simulink model "WLTP"  (R2020b)
settings: Solver=FixedStepAuto  StartTime=0.0  StopTime=1800  FixedStep=1  RelTol=1e-3
values from neighbouring files (symbols this model uses):
  A = 2.4    [Ansteuerung_WLTP.m]
  cw = 0.28    [Ansteuerung_WLTP.m]
  eta = VKM.eta    [Ansteuerung_WLTP.m]
  eta_diff = 0.99    [Ansteuerung_WLTP.m]
  eta_getr = 0.96    [Ansteuerung_WLTP.m]
  Fr = 40    [Ansteuerung_WLTP.m]
  fr = 1e-3    (= 0.001)    [Ansteuerung_WLTP.m]
  g = 9.81    [Ansteuerung_WLTP.m]
  i = [4.776 3.360 2.311 1.553 1.020 0.655]    [Ansteuerung_WLTP.m]
  i_AG = 3.825    [Ansteuerung_WLTP.m]
  lambda = 1.25    [Ansteuerung_WLTP.m]
  M_1 = eta_diff*eta_getr*VKM.full_load_M*i(1)*i_AG    [Ansteuerung_WLTP.m]
  M_2 = eta_diff*eta_getr*VKM.full_load_M*i(2)*i_AG    [Ansteuerung_WLTP.m]
  M_3 = eta_diff*eta_getr*VKM.full_load_M*i(3)*i_AG    [Ansteuerung_WLTP.m]
  M_4 = eta_diff*eta_getr*VKM.full_load_M*i(4)*i_AG    [Ansteuerung_WLTP.m]
  M_5 = eta_diff*eta_getr*VKM.full_load_M*i(5)*i_AG    [Ansteuerung_WLTP.m]
  M_6 = eta_diff*eta_getr*VKM.full_load_M*i(6)*i_AG    [Ansteuerung_WLTP.m]
  mfzg = 1500    [Ansteuerung_WLTP.m]
  mzul = 475    [Ansteuerung_WLTP.m]
  n_u = 900    [Ansteuerung_WLTP.m]
  rdyn = 0.35    [Ansteuerung_WLTP.m]
  rho = 1.2    [Ansteuerung_WLTP.m]
  v1_1 = (pi*VKM.full_load_n*rdyn)*3.6/(30*i_AG*i(1))    [Ansteuerung_WLTP.m]
  v1_2 = (pi*VKM.full_load_n*rdyn)*3.6/(30*i_AG*i(2))    [Ansteuerung_WLTP.m]
  v1_3 = (pi*VKM.full_load_n*rdyn)*3.6/(30*i_AG*i(3))    [Ansteuerung_WLTP.m]
  v1_4 = (pi*VKM.full_load_n*rdyn)*3.6/(30*i_AG*i(4))    [Ansteuerung_WLTP.m]
  v1_5 = (pi*VKM.full_load_n*rdyn)*3.6/(30*i_AG*i(5))    [Ansteuerung_WLTP.m]
  v1_6 = (pi*VKM.full_load_n*rdyn)*3.6/(30*i_AG*i(6))    [Ansteuerung_WLTP.m]
  VKM =     [VKM.mat]
  WLTP_t = [0:1800].'    [Ansteuerung_WLTP.m]
  WLTP_v = [0;0;0;0;0;0;0;0;0;0;0;0;0.200000000000000;1.70000000000000;5.40000000000000;9.90000000000000;13.1000000000000;16.9000000000000;21.7000000000000;26;27.5000000000000;28.1000000000000;28.3000000000000;28.8000000000000;29.1000000000000;30.8000000000000;31.9000000000000;34.1000000000000;36.6000000000000;39.1000000000000;41.3000000000000;42.5000000000000;43.3000000000000;43.9000000000000;44.40000000000 ...(+23900 chars)    [Ansteuerung_WLTP.m]
settings Model: Creator=ohms  LastModifiedBy=kusno

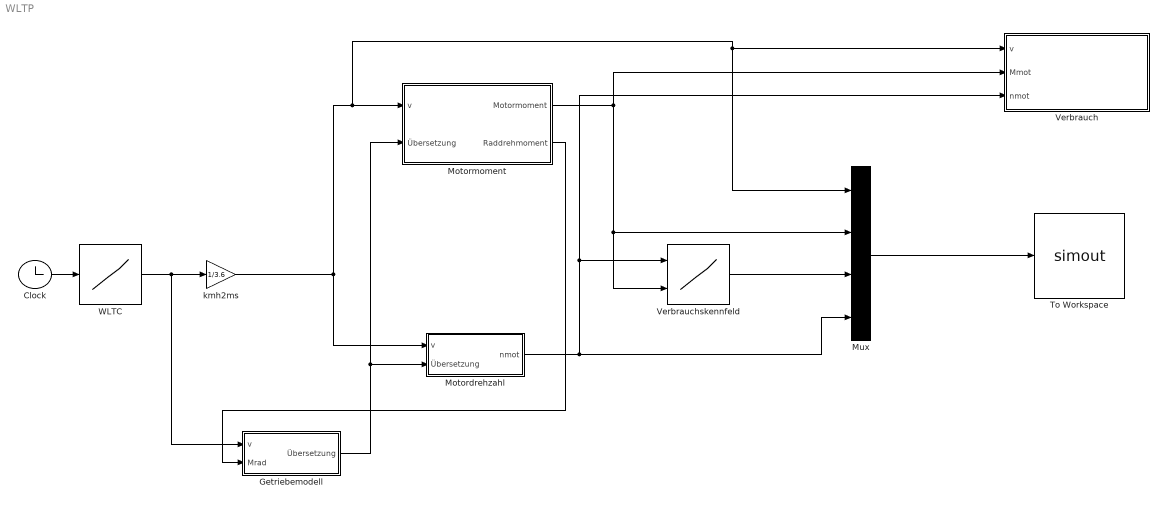
== system WLTP ==
  Clock : Clock
  Getriebemodell : Subsystem
  Motordrehzahl : Subsystem
  Motormoment : Subsystem
  Mux : Mux
  To Workspace : ToWorkspace  VariableName=simout  SaveFormat=Timeseries  SampleTime=-1
  Verbrauch : Subsystem
  Verbrauchskennfeld : Lookup_n-D  BreakpointsForDimension1=VKM.n_axis(:,1)  BreakpointsForDimension2=VKM.M_axis(1,:)  Table=eta  ExtrapMethod=Clip  InternalRulePriority=Speed  RndMeth=Simplest  InputSameDT=on
      settings: InputPortMap=u0,u1
  WLTC : Lookup_n-D  NumberOfTableDimensions=1  BreakpointsForDimension1=WLTP_t  Table=WLTP_v  InternalRulePriority=Speed  RndMeth=Simplest  InputSameDT=on
  kmh2ms : Gain  Gain=1/3.6
  wires:
  Clock/1 -> WLTC/1
  Getriebemodell/1(Übersetzung) -> Motormoment/2(Übersetzung), Motordrehzahl/2(Übersetzung)
  kmh2ms/1 -> Motormoment/1(v), Mux/1, Verbrauch/1(v), Motordrehzahl/1(v)
  Motordrehzahl/1(nmot) -> Verbrauch/3(nmot), Verbrauchskennfeld/1, Mux/4
  Mux/1 -> To Workspace/1
  Motormoment/1(Motormoment) -> Mux/2, Verbrauchskennfeld/2, Verbrauch/2(Mmot)
  Verbrauchskennfeld/1 -> Mux/3
  Motormoment/2(Raddrehmoment) -> Getriebemodell/2(Mrad)
  WLTC/1 -> Getriebemodell/1(v), kmh2ms/1

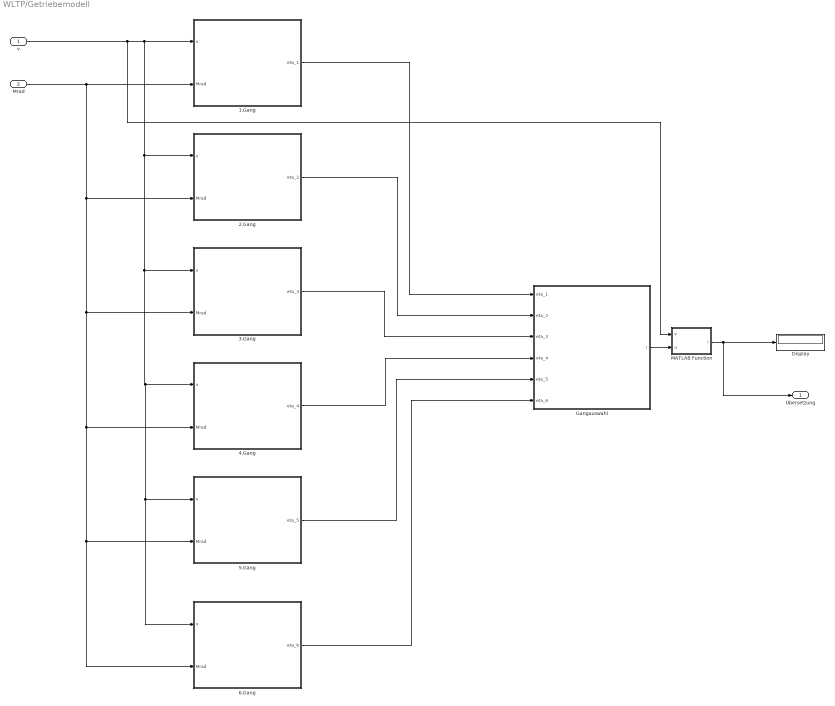
== system WLTP/Getriebemodell ==
  v : Inport
  Mrad : Inport  Port=2
  1.Gang : Subsystem
  2.Gang : Subsystem
  3.Gang : Subsystem
  4.Gang : Subsystem
  5.Gang : Subsystem
  6.Gang : Subsystem
  Display : Display
  Gangauswahl : MATLAB Function  TreatAsAtomicUnit=on
  MATLAB Function : MATLAB Function  TreatAsAtomicUnit=on
  Übersetzung : Outport
  wires:
  Mrad/1 -> 6.Gang/2(Mrad), 5.Gang/2(Mrad), 4.Gang/2(Mrad), 3.Gang/2(Mrad), 2.Gang/2(Mrad), 1.Gang/2(Mrad)
  1.Gang/1(eta_1) -> Gangauswahl/1(eta_1)
  2.Gang/1(eta_2) -> Gangauswahl/2(eta_2)
  3.Gang/1(eta_3) -> Gangauswahl/3(eta_3)
  4.Gang/1(eta_4) -> Gangauswahl/4(eta_4)
  5.Gang/1(eta_5) -> Gangauswahl/5(eta_5)
  6.Gang/1(eta_6) -> Gangauswahl/6(eta_6)
  Gangauswahl/1(i) -> MATLAB Function/2(u)
  MATLAB Function/1(i) -> Display/1, Übersetzung/1
  v/1 -> MATLAB Function/1(v), 6.Gang/1(v), 5.Gang/1(v), 4.Gang/1(v), 3.Gang/1(v), 2.Gang/1(v), 1.Gang/1(v)

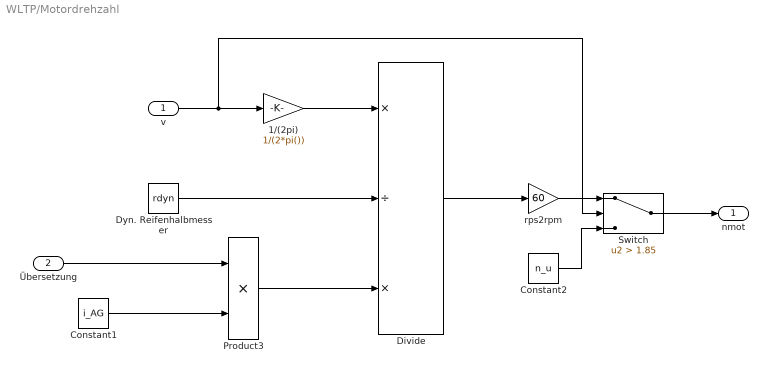
== system WLTP/Motordrehzahl ==
  v : Inport
  Übersetzung : Inport  Port=2
  1/(2pi) : Gain  Gain=1/(2*pi())
  Constant1 : Constant  Value=i_AG
  Constant2 : Constant  Value=n_u
  Divide : Product  Inputs=*/*
  Dyn. Reifenhalbmesser : Constant  Value=rdyn
  Product3 : Product
  Switch : Switch  Criteria=u2 > Threshold  Threshold=1.85
  rps2rpm : Gain  Gain=60
  nmot : Outport
  wires:
  v/1 -> Switch/2, 1/(2pi)/1
  1/(2pi)/1 -> Divide/1
  Dyn. Reifenhalbmesser/1 -> Divide/2
  Divide/1 -> rps2rpm/1
  Übersetzung/1 -> Product3/1
  Constant1/1 -> Product3/2
  Product3/1 -> Divide/3
  Switch/1 -> nmot/1
  rps2rpm/1 -> Switch/1
  Constant2/1 -> Switch/3

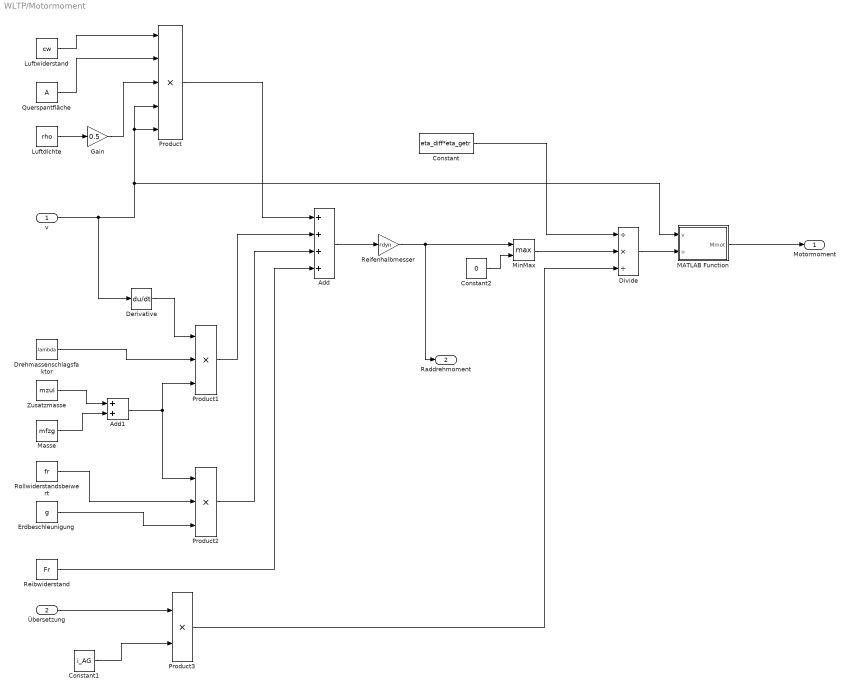
== system WLTP/Motormoment ==
  v : Inport
  Übersetzung : Inport  Port=2
  Add : Sum  Inputs=++++
  Add1 : Sum
  Constant : Constant  Value=eta_diff*eta_getr
  Constant1 : Constant  Value=i_AG
  Constant2 : Constant  Value=0
  Derivative : Derivative
  Divide : Product  Inputs=/*/
  Drehmassenschlagsfaktor : Constant  Value=lambda
  Erdbeschleunigung : Constant  Value=g
  Gain : Gain  Gain=0.5
  Luftdichte : Constant  Value=rho
  Luftwiderstand : Constant  Value=cw
  MATLAB Function : MATLAB Function  TreatAsAtomicUnit=on
  Masse : Constant  Value=mfzg
  MinMax : MinMax  Function=max  Inputs=2
  Product : Product  Inputs=5
  Product1 : Product  Inputs=3
  Product2 : Product  Inputs=3
  Product3 : Product
  Querspantfläche : Constant  Value=A
  Reibwiderstand : Constant  Value=Fr
  Reifenhalbmesser : Gain  Gain=rdyn
  Rollwiderstandsbeiwert : Constant  Value=fr
  Zusatzmasse : Constant  Value=mzul
  Motormoment : Outport
  Raddrehmoment : Outport  Port=2
  wires:
  Luftwiderstand/1 -> Product/1
  Querspantfläche/1 -> Product/2
  Luftdichte/1 -> Gain/1
  Gain/1 -> Product/3
  Derivative/1 -> Product1/1
  Drehmassenschlagsfaktor/1 -> Product1/2
  Rollwiderstandsbeiwert/1 -> Product2/2
  Erdbeschleunigung/1 -> Product2/3
  v/1 -> Derivative/1, MATLAB Function/1(v), Product/5, Product/4
  Product/1 -> Add/1
  Product1/1 -> Add/2
  Product2/1 -> Add/3
  Reifenhalbmesser/1 -> MinMax/1, Raddrehmoment/1
  Reibwiderstand/1 -> Add/4
  Constant/1 -> Divide/1
  Übersetzung/1 -> Product3/1
  Constant1/1 -> Product3/2
  Product3/1 -> Divide/3
  Add/1 -> Reifenhalbmesser/1
  Divide/1 -> MATLAB Function/2(u)
  MATLAB Function/1(Mmot) -> Motormoment/1
  Zusatzmasse/1 -> Add1/1
  Masse/1 -> Add1/2
  Add1/1 -> Product1/3, Product2/1
  MinMax/1 -> Divide/2
  Constant2/1 -> MinMax/2

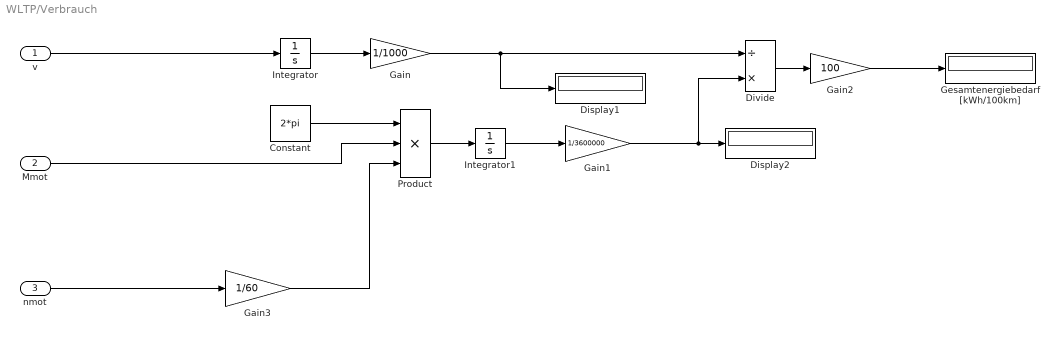
== system WLTP/Verbrauch ==
  v : Inport
  Mmot : Inport  Port=2
  nmot : Inport  Port=3
  Constant : Constant  Value=2*pi
  Display1 : Display
  Display2 : Display
  Divide : Product  Inputs=/*
  Gain : Gain  Gain=1/1000
  Gain1 : Gain  Gain=1/3600000
  Gain2 : Gain  Gain=100
  Gain3 : Gain  Gain=1/60
  Gesamtenergiebedarf [kWh/100km] : Display
  Integrator : Integrator
  Integrator1 : Integrator
  Product : Product  Inputs=3
  wires:
  Gain1/1 -> Display2/1, Divide/2
  Mmot/1 -> Product/2
  Integrator/1 -> Gain/1
  Divide/1 -> Gain2/1
  v/1 -> Integrator/1
  Gain/1 -> Display1/1, Divide/1
  Product/1 -> Integrator1/1
  Constant/1 -> Product/1
  nmot/1 -> Gain3/1
  Gain2/1 -> Gesamtenergiebedarf [kWh/100km]/1
  Integrator1/1 -> Gain1/1
  Gain3/1 -> Product/3

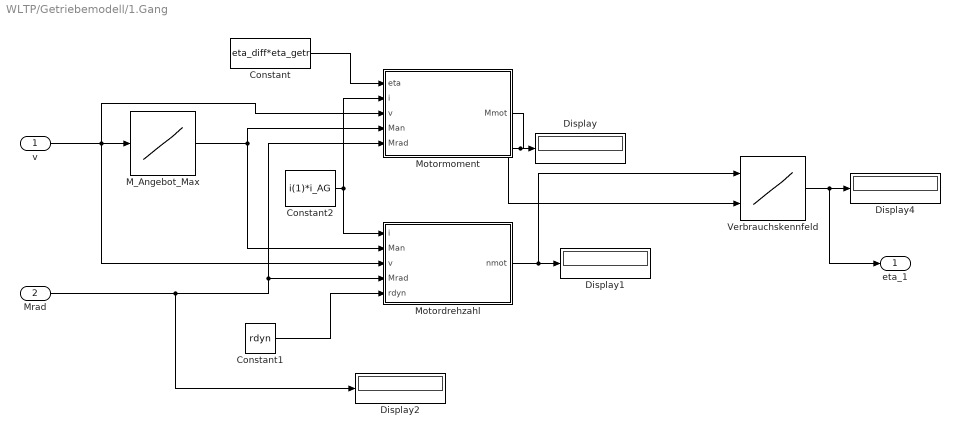
== system WLTP/Getriebemodell/1.Gang ==
  v : Inport
  Mrad : Inport  Port=2
  Constant : Constant  Value=eta_diff*eta_getr
  Constant1 : Constant  Value=rdyn
  Constant2 : Constant  Value=i(1)*i_AG
  Display{,1..2,4} (4 alike) : Display
  M_Angebot_Max : Lookup_n-D  NumberOfTableDimensions=1  BreakpointsForDimension1=v1_1  Table=M_1  InternalRulePriority=Speed  RndMeth=Simplest  InputSameDT=on
  Motordrehzahl : MATLAB Function  TreatAsAtomicUnit=on
  Motormoment : MATLAB Function  TreatAsAtomicUnit=on
  Verbrauchskennfeld : Lookup_n-D  BreakpointsForDimension1=VKM.n_axis(:,1)  BreakpointsForDimension2=VKM.M_axis(1,:)  Table=eta  ExtrapMethod=Clip  InternalRulePriority=Speed  RndMeth=Simplest  InputSameDT=on
      settings: InputPortMap=u0,u1
  eta_1 : Outport
  wires:
  v/1 -> Motordrehzahl/3(v), Motormoment/3(v), M_Angebot_Max/1
  Mrad/1 -> Display2/1, Motordrehzahl/4(Mrad), Motormoment/5(Mrad)
  Motormoment/1(Mmot) -> Verbrauchskennfeld/2, Display/1
  Constant2/1 -> Motordrehzahl/1(i), Motormoment/2(i)
  Constant1/1 -> Motordrehzahl/5(rdyn)
  Motordrehzahl/1(nmot) -> Verbrauchskennfeld/1, Display1/1
  Verbrauchskennfeld/1 -> eta_1/1, Display4/1
  Constant/1 -> Motormoment/1(eta)
  M_Angebot_Max/1 -> Motordrehzahl/2(Man), Motormoment/4(Man)

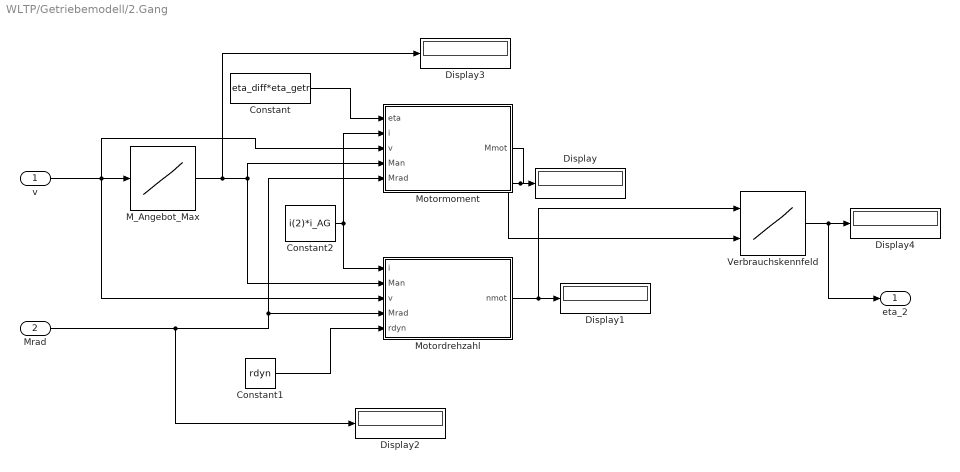
== system WLTP/Getriebemodell/2.Gang ==
  v : Inport
  Mrad : Inport  Port=2
  Constant : Constant  Value=eta_diff*eta_getr
  Constant1 : Constant  Value=rdyn
  Constant2 : Constant  Value=i(2)*i_AG
  Display{,1..4} (5 alike) : Display
  M_Angebot_Max : Lookup_n-D  NumberOfTableDimensions=1  BreakpointsForDimension1=v1_2  Table=M_2  InternalRulePriority=Speed  RndMeth=Simplest  InputSameDT=on
  Motordrehzahl : MATLAB Function  TreatAsAtomicUnit=on
  Motormoment : MATLAB Function  TreatAsAtomicUnit=on
  Verbrauchskennfeld : Lookup_n-D  BreakpointsForDimension1=VKM.n_axis(:,1)  BreakpointsForDimension2=VKM.M_axis(1,:)  Table=eta  ExtrapMethod=Clip  InternalRulePriority=Speed  RndMeth=Simplest  InputSameDT=on
      settings: InputPortMap=u0,u1
  eta_2 : Outport
  wires:
  v/1 -> Motordrehzahl/3(v), Motormoment/3(v), M_Angebot_Max/1
  M_Angebot_Max/1 -> Display3/1, Motordrehzahl/2(Man), Motormoment/4(Man)
  Mrad/1 -> Display2/1, Motordrehzahl/4(Mrad), Motormoment/5(Mrad)
  Motormoment/1(Mmot) -> Verbrauchskennfeld/2, Display/1
  Constant2/1 -> Motordrehzahl/1(i), Motormoment/2(i)
  Constant1/1 -> Motordrehzahl/5(rdyn)
  Motordrehzahl/1(nmot) -> Verbrauchskennfeld/1, Display1/1
  Constant/1 -> Motormoment/1(eta)
  Verbrauchskennfeld/1 -> eta_2/1, Display4/1

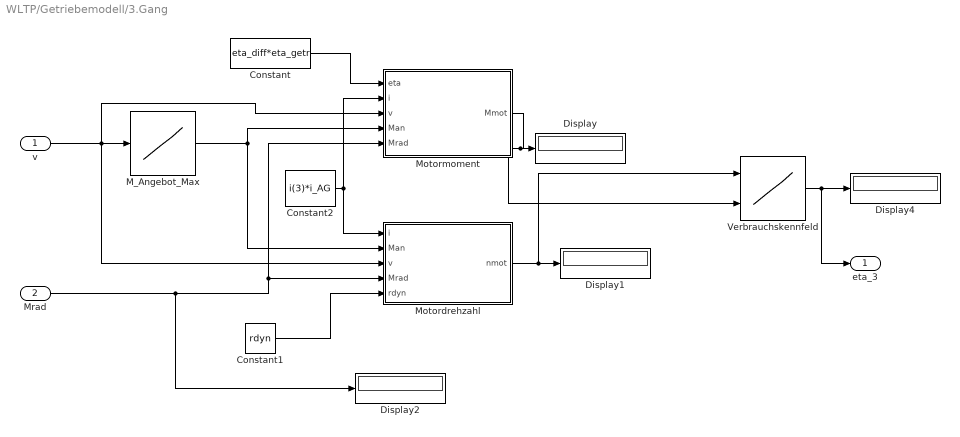
== system WLTP/Getriebemodell/3.Gang ==
  v : Inport
  Mrad : Inport  Port=2
  Constant : Constant  Value=eta_diff*eta_getr
  Constant1 : Constant  Value=rdyn
  Constant2 : Constant  Value=i(3)*i_AG
  Display{,1..2,4} (4 alike) : Display
  M_Angebot_Max : Lookup_n-D  NumberOfTableDimensions=1  BreakpointsForDimension1=v1_3  Table=M_3  InternalRulePriority=Speed  RndMeth=Simplest  InputSameDT=on
  Motordrehzahl : MATLAB Function  TreatAsAtomicUnit=on
  Motormoment : MATLAB Function  TreatAsAtomicUnit=on
  Verbrauchskennfeld : Lookup_n-D  BreakpointsForDimension1=VKM.n_axis(:,1)  BreakpointsForDimension2=VKM.M_axis(1,:)  Table=eta  ExtrapMethod=Clip  InternalRulePriority=Speed  RndMeth=Simplest  InputSameDT=on
      settings: InputPortMap=u0,u1
  eta_3 : Outport
  wires:
  v/1 -> Motordrehzahl/3(v), Motormoment/3(v), M_Angebot_Max/1
  Mrad/1 -> Display2/1, Motordrehzahl/4(Mrad), Motormoment/5(Mrad)
  Motormoment/1(Mmot) -> Verbrauchskennfeld/2, Display/1
  Constant2/1 -> Motordrehzahl/1(i), Motormoment/2(i)
  Constant1/1 -> Motordrehzahl/5(rdyn)
  Motordrehzahl/1(nmot) -> Verbrauchskennfeld/1, Display1/1
  Verbrauchskennfeld/1 -> eta_3/1, Display4/1
  Constant/1 -> Motormoment/1(eta)
  M_Angebot_Max/1 -> Motordrehzahl/2(Man), Motormoment/4(Man)

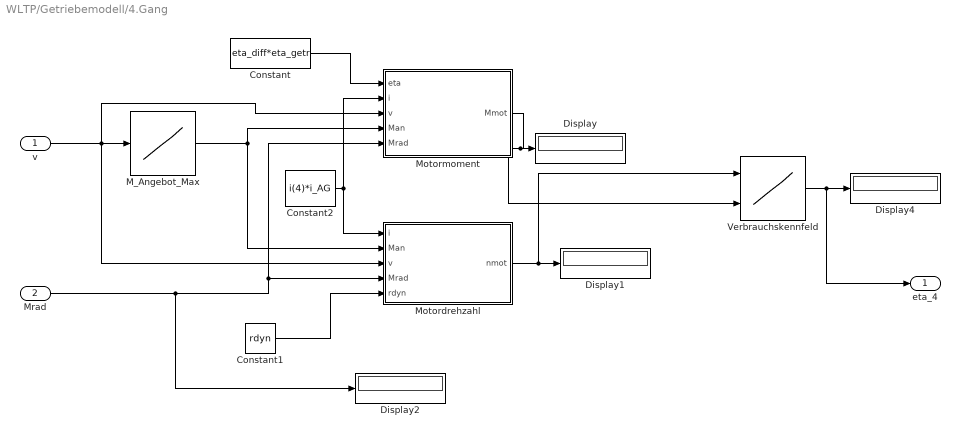
== system WLTP/Getriebemodell/4.Gang ==
  v : Inport
  Mrad : Inport  Port=2
  Constant : Constant  Value=eta_diff*eta_getr
  Constant1 : Constant  Value=rdyn
  Constant2 : Constant  Value=i(4)*i_AG
  Display{,1..2,4} (4 alike) : Display
  M_Angebot_Max : Lookup_n-D  NumberOfTableDimensions=1  BreakpointsForDimension1=v1_4  Table=M_4  InternalRulePriority=Speed  RndMeth=Simplest  InputSameDT=on
  Motordrehzahl : MATLAB Function  TreatAsAtomicUnit=on
  Motormoment : MATLAB Function  TreatAsAtomicUnit=on
  Verbrauchskennfeld : Lookup_n-D  BreakpointsForDimension1=VKM.n_axis(:,1)  BreakpointsForDimension2=VKM.M_axis(1,:)  Table=eta  ExtrapMethod=Clip  InternalRulePriority=Speed  RndMeth=Simplest  InputSameDT=on
      settings: InputPortMap=u0,u1
  eta_4 : Outport
  wires:
  v/1 -> Motordrehzahl/3(v), Motormoment/3(v), M_Angebot_Max/1
  M_Angebot_Max/1 -> Motordrehzahl/2(Man), Motormoment/4(Man)
  Mrad/1 -> Display2/1, Motordrehzahl/4(Mrad), Motormoment/5(Mrad)
  Motormoment/1(Mmot) -> Verbrauchskennfeld/2, Display/1
  Constant2/1 -> Motordrehzahl/1(i), Motormoment/2(i)
  Constant1/1 -> Motordrehzahl/5(rdyn)
  Motordrehzahl/1(nmot) -> Verbrauchskennfeld/1, Display1/1
  Constant/1 -> Motormoment/1(eta)
  Verbrauchskennfeld/1 -> eta_4/1, Display4/1

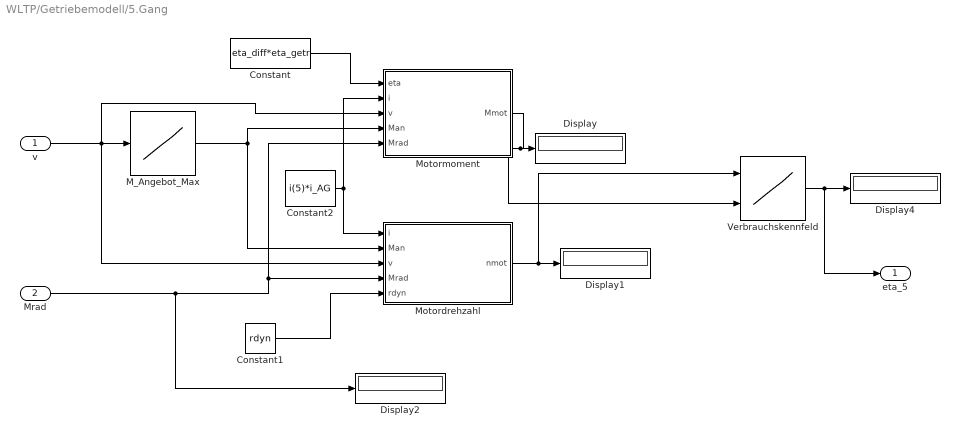
== system WLTP/Getriebemodell/5.Gang ==
  v : Inport
  Mrad : Inport  Port=2
  Constant : Constant  Value=eta_diff*eta_getr
  Constant1 : Constant  Value=rdyn
  Constant2 : Constant  Value=i(5)*i_AG
  Display{,1..2,4} (4 alike) : Display
  M_Angebot_Max : Lookup_n-D  NumberOfTableDimensions=1  BreakpointsForDimension1=v1_5  Table=M_5  InternalRulePriority=Speed  RndMeth=Simplest  InputSameDT=on
  Motordrehzahl : MATLAB Function  TreatAsAtomicUnit=on
  Motormoment : MATLAB Function  TreatAsAtomicUnit=on
  Verbrauchskennfeld : Lookup_n-D  BreakpointsForDimension1=VKM.n_axis(:,1)  BreakpointsForDimension2=VKM.M_axis(1,:)  Table=eta  ExtrapMethod=Clip  InternalRulePriority=Speed  RndMeth=Simplest  InputSameDT=on
      settings: InputPortMap=u0,u1
  eta_5 : Outport
  wires:
  v/1 -> Motordrehzahl/3(v), Motormoment/3(v), M_Angebot_Max/1
  M_Angebot_Max/1 -> Motordrehzahl/2(Man), Motormoment/4(Man)
  Mrad/1 -> Display2/1, Motordrehzahl/4(Mrad), Motormoment/5(Mrad)
  Motormoment/1(Mmot) -> Verbrauchskennfeld/2, Display/1
  Constant2/1 -> Motordrehzahl/1(i), Motormoment/2(i)
  Constant1/1 -> Motordrehzahl/5(rdyn)
  Motordrehzahl/1(nmot) -> Verbrauchskennfeld/1, Display1/1
  Verbrauchskennfeld/1 -> eta_5/1, Display4/1
  Constant/1 -> Motormoment/1(eta)

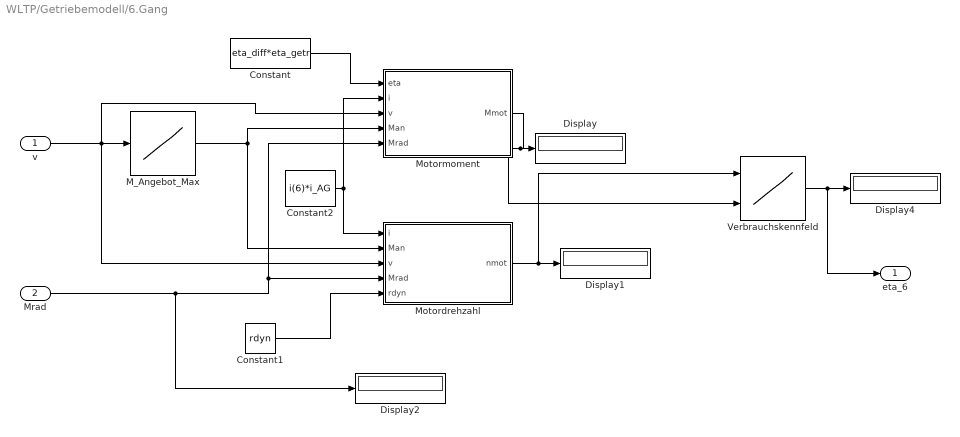
== system WLTP/Getriebemodell/6.Gang ==
  v : Inport
  Mrad : Inport  Port=2
  Constant : Constant  Value=eta_diff*eta_getr
  Constant1 : Constant  Value=rdyn
  Constant2 : Constant  Value=i(6)*i_AG
  Display{,1..2,4} (4 alike) : Display
  M_Angebot_Max : Lookup_n-D  NumberOfTableDimensions=1  BreakpointsForDimension1=v1_6  Table=M_6  InternalRulePriority=Speed  RndMeth=Simplest  InputSameDT=on
  Motordrehzahl : MATLAB Function  TreatAsAtomicUnit=on
  Motormoment : MATLAB Function  TreatAsAtomicUnit=on
  Verbrauchskennfeld : Lookup_n-D  BreakpointsForDimension1=VKM.n_axis(:,1)  BreakpointsForDimension2=VKM.M_axis(1,:)  Table=eta  ExtrapMethod=Clip  InternalRulePriority=Speed  RndMeth=Simplest  InputSameDT=on
      settings: InputPortMap=u0,u1
  eta_6 : Outport
  wires:
  v/1 -> Motordrehzahl/3(v), Motormoment/3(v), M_Angebot_Max/1
  M_Angebot_Max/1 -> Motordrehzahl/2(Man), Motormoment/4(Man)
  Mrad/1 -> Display2/1, Motordrehzahl/4(Mrad), Motormoment/5(Mrad)
  Motormoment/1(Mmot) -> Verbrauchskennfeld/2, Display/1
  Constant2/1 -> Motordrehzahl/1(i), Motormoment/2(i)
  Constant1/1 -> Motordrehzahl/5(rdyn)
  Motordrehzahl/1(nmot) -> Verbrauchskennfeld/1, Display1/1
  Verbrauchskennfeld/1 -> eta_6/1, Display4/1
  Constant/1 -> Motormoment/1(eta)

== matlab function WLTP/Getriebemodell/5.Gang/Motordrehzahl ==
  data: i input; Man input; v input; nmot output; Mrad input; rdyn input
function nmot = fcn(i, Man,v , Mrad, rdyn)
%Man : Angebotsdrehmoment vom Rad(Abhängig von v und i)
%Mrad : Aktuelle Raddrehmoment

if (30.437575882530865<=v) && (v<=(2.029171725502058e+02)) && (Mrad<Man)
    nmot =v*i*30/(rdyn*pi()*3.6);
else
    nmot=0;


end

== matlab function WLTP/Getriebemodell/5.Gang/Motormoment ==
  data: eta input; i input; v input; Man input; Mmot output; Mrad input
function Mmot = fcn(eta, i, v, Man, Mrad)

%Man : Angebotsdrehmoment vom Rad(Abhängig von v und i)
%Mrad : Aktuelle Raddrehmoment

if (30.437575882530865<=v) && (v<=(2.029171725502058e+02)) && (Mrad<Man)
    Mmot =Mrad/(i*eta);
else
     Mmot=0;
    

end

== matlab function WLTP/Getriebemodell/6.Gang/Motordrehzahl ==
  data: i input; Man input; v input; nmot output; Mrad input; rdyn input
function nmot = fcn(i, Man,v , Mrad, rdyn)
%Man : Angebotsdrehmoment vom Rad(Abhängig von v und i)
%Mrad : Aktuelle Raddrehmoment

if (47.398973130048060<=v) && (v<=(3.159931542003204e+02)) && (Mrad<Man)
    nmot =v*i*30/(rdyn*pi()*3.6);
else
    nmot=0;


end

== matlab function WLTP/Getriebemodell/6.Gang/Motormoment ==
  data: eta input; i input; v input; Man input; Mmot output; Mrad input
function Mmot = fcn(eta, i, v, Man, Mrad)

%Man : Angebotsdrehmoment vom Rad(Abhängig von v und i)
%Mrad : Aktuelle Raddrehmoment

if (47.398973130048060<=v) && (v<=(3.159931542003204e+02)) && (Mrad<Man)
    Mmot =Mrad/(i*eta);
else
     Mmot=0;
    

end

== matlab function WLTP/Getriebemodell/Gangauswahl ==
  data: eta_1 input; eta_2 input; i output; eta_3 input; eta_4 input; eta_5 input; eta_6 input
function i = fcn(eta_1, eta_2, eta_3, eta_4, eta_5, eta_6)

eta_wahl=[eta_1 eta_2 eta_3 eta_4 eta_5 eta_6];
Max=max(eta_wahl);

if (Max==eta_1)
    i=4.776;
     elseif (Max==eta_2)
          i=3.360;
              elseif (Max==eta_3)
                  i=2.311;
                      elseif (Max==eta_4)
                        i=1.553;
                             elseif (Max==eta_5)
                                 i=1.020;
                                  elseif (Max==eta_6)
                                     i=0.655;
                      
else i=0;
        
   
end

== matlab function WLTP/Motormoment/MATLAB Function ==
  data: v input; u input; Mmot output
function Mmot = fcn(v,u)
if v==0
    Mmot=0;
else
Mmot = u;
end

== matlab function WLTP/Getriebemodell/MATLAB Function ==
  data: v input; u input; i output
function i = fcn(v,u)
if (v==0) | (v<6.500487311595789)
    i = 4.776;
else
    i=u;
end

== matlab function WLTP/Getriebemodell/1.Gang/Motordrehzahl ==
  data: i input; Man input; v input; nmot output; Mrad input; rdyn input
function nmot = fcn(i, Man,v , Mrad, rdyn)
%Man : Angebotsdrehmoment vom Rad(Abhängig von v und i)
%Mrad : Aktuelle Raddrehmoment

if (v<=43.336582077305260) && (Mrad<Man)
    nmot =v*i*30/(rdyn*pi()*3.6);
else
    nmot=0;


end

== matlab function WLTP/Getriebemodell/1.Gang/Motormoment ==
  data: eta input; i input; v input; Man input; Mmot output; Mrad input
function Mmot = fcn(eta, i, v, Man, Mrad)

%Man : Angebotsdrehmoment vom Rad(Abhängig von v und i)
%Mrad : Aktuelle Raddrehmoment

if (v<=43.336582077305260) && (Mrad<Man)
    Mmot =Mrad/(i*eta);
else
     Mmot=0;
    

end

== matlab function WLTP/Getriebemodell/2.Gang/Motordrehzahl ==
  data: i input; Man input; v input; nmot output; Mrad input; rdyn input
function nmot = fcn(i, Man,v , Mrad, rdyn)
%Man : Angebotsdrehmoment vom Rad(Abhängig von v und i)
%Mrad : Aktuelle Raddrehmoment

if (9.239978392911157<=v) && (v<=61.599855952741040) && (Mrad<Man)
    nmot =v*i*30/(rdyn*pi()*3.6);
else
    nmot=0;


end

== matlab function WLTP/Getriebemodell/2.Gang/Motormoment ==
  data: eta input; i input; v input; Man input; Mmot output; Mrad input
function Mmot = fcn(eta, i, v, Man, Mrad)

%Man : Angebotsdrehmoment vom Rad(Abhängig von v und i)
%Mrad : Aktuelle Raddrehmoment

if (9.239978392911157<=v) && (v<=61.599855952741040) && (Mrad<Man)
    Mmot =Mrad/(i*eta);
else
     Mmot=0;
    

end

== matlab function WLTP/Getriebemodell/3.Gang/Motordrehzahl ==
  data: i input; Man input; v input; nmot output; Mrad input; rdyn input
function nmot = fcn(i, Man,v , Mrad, rdyn)
%Man : Angebotsdrehmoment vom Rad(Abhängig von v und i)
%Mrad : Aktuelle Raddrehmoment

if (13.434152920892030<=v) && (v<=89.561019472613540) && (Mrad<Man)
    nmot =v*i*30/(rdyn*pi()*3.6);
else
    nmot=0;


end

== matlab function WLTP/Getriebemodell/3.Gang/Motormoment ==
  data: eta input; i input; v input; Man input; Mmot output; Mrad input
function Mmot = fcn(eta, i, v, Man, Mrad)

%Man : Angebotsdrehmoment vom Rad(Abhängig von v und i)
%Mrad : Aktuelle Raddrehmoment

if (13.434152920892030<=v) && (v<=89.561019472613540) && (Mrad<Man)
    Mmot =Mrad/(i*eta);
else
     Mmot=0;
    

end

== matlab function WLTP/Getriebemodell/4.Gang/Motordrehzahl ==
  data: i input; Man input; v input; nmot output; Mrad input; rdyn input
function nmot = fcn(i, Man,v , Mrad, rdyn)
%Man : Angebotsdrehmoment vom Rad(Abhängig von v und i)
%Mrad : Aktuelle Raddrehmoment

if (19.991196007843840<=v) && (v<=(1.332746400522923e+02)) && (Mrad<Man)
    nmot =v*i*30/(rdyn*pi()*3.6);
else
    nmot=0;


end

== matlab function WLTP/Getriebemodell/4.Gang/Motormoment ==
  data: eta input; i input; v input; Man input; Mmot output; Mrad input
function Mmot = fcn(eta, i, v, Man, Mrad)

%Man : Angebotsdrehmoment vom Rad(Abhängig von v und i)
%Mrad : Aktuelle Raddrehmoment

if (19.991196007843840<=v) && (v<=(1.332746400522923e+02)) && (Mrad<Man)
    Mmot =Mrad/(i*eta);
else
     Mmot=0;
    

end
